simulink model "chap1_3_org"  (Simulink 10.0)
settings: Solver=ode45  StartTime=0.0  StopTime=10.0  RelTol=1e-3  EnableMultiTasking=on
settings Model: Creator=Administrator  LastModifiedBy=bhisma
settings DataIOCC: LimitDataPoints=on
settings OptimizationCC: ExpressionDepthLimit=2147483647
settings DebuggingCC: SolverPrmCheckMsg=warning  StateNameClashWarn=warning
settings GRTTargetCC: GeneratePreprocessorConditionals=Disable all  CombineOutputUpdateFcns=on  GRTInterface=off
settings ConfigComp: CovExternalEMLEnable=off

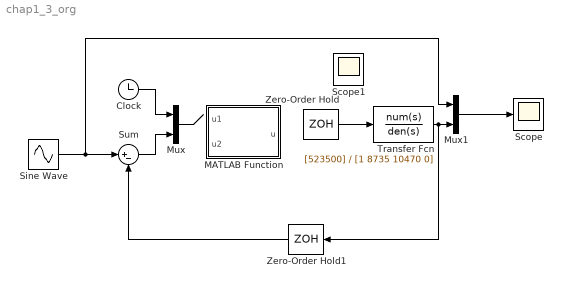
== system chap1_3_org ==
  Clock : Clock
  MATLAB Function : MATLAB Function  TreatAsAtomicUnit=on
  Mux : Mux  Inputs=2
  Mux1 : Mux  Inputs=2
  Scope : Scope
  Scope1 : Scope
  Sine Wave : Sin  SampleTime=0.001
  Sum : Sum  Inputs=|+-
  Transfer Fcn : TransferFcn  Numerator=[523500]  Denominator=[1 8735 10470 0]
  Zero-Order Hold : ZeroOrderHold
  Zero-Order Hold1 : ZeroOrderHold
  wires:
  Clock/1 -> Mux/1
  Sum/1 -> Mux/2
  Sine Wave/1 -> Mux1/1, Sum/1
  Mux/1 -> ?
  Transfer Fcn/1 -> Zero-Order Hold1/1, Mux1/2
  Mux1/1 -> Scope/1
  ? -> Scope1/1, Zero-Order Hold/1
  Zero-Order Hold/1 -> Transfer Fcn/1
  Zero-Order Hold1/1 -> Sum/2

== matlab function MATLAB Function ==
  data: u output double; u1 input double; u2 input double
function u  = pidsimf(u1,u2)
%#codegen
persistent pidmat errori error_1
if u1==0
    errori=0;
    error_l=0;
end
ts=0.001;
kp=1.5;
ki=2.0;
kd=0.05;

error=u2;
errori=errori+error*ts;
errord=(error-error_l)/ts;

u=kp*error+ki*errori+kd*errord;
error_l=error;
